simulink model "Demo_PreScanCarSim3D_FMU_cs"  (Simulink 8.6)
settings: Solver=ode5  SolverMode=SingleTasking  StartTime=0.0  StopTime=68  FixedStep=1/1000  RelTol=1e-3
PreLoadFcn:
  | mbxruntime.callbacks.PreLoadFcn(bdroot);
  | check_NUTS_defined;
  | 
  | assignin('base',['model_closed_' bdroot],false);
PostLoadFcn:
  | mbxruntime.callbacks.PostLoadFcn(bdroot);
InitFcn:
  | mbxruntime.callbacks.InitFcn(bdroot);
StartFcn:
  | mbxruntime.callbacks.StartFcn(bdroot);
StopFcn:
  | mbxruntime.callbacks.StopFcn(bdroot);
undefined symbols (not defined in the file or in its folder): DiscIntNeverNeededParam, mbxruntime, tabledata, warningInitialVelocity, x0, x_ini_VRML, y_ini_VRML, z_ini_VRML
libraries: PreScanSimulinkLibrary x15, simulink_extras x8, simulink x5, PreScanCarSimLibrary x1, fmu_cs_lib x1
(part 5 of 11)

== system Demo_PreScanCarSim3D_FMU_cs/VISUCasingLights_TrafficLightRoadSideNL_1/ENABLED/Actuator ==
  VISUCasingLights_TrafficLightRoadSideNL_1 : Inport  Tag=inport/VisuCasingLights  SampleTime=50/1000  BusOutputAsStruct=on
  DemuxVisuLights : Demux  Outputs=3
  LimiterVisuLights : Saturate  UpperLimit=1  LowerLimit=0
  visu_Green [-] : S-Function  FunctionName=sfun_MaterialColorSelector  Parameters=mbxruntime.parameters.convert(UniqueID), mbxruntime.parameters.convert(ColorsObjectQuery), mbxruntime.parameters.convert(Colors),tabledata, TimeStep  SFunctionDeploymentMode=off  EnableBusSupport=off  mask(PreScan Sink Block: VisuTrafficLight){UniqueID=2553, ColorsObjectQuery=child:name=TrafficLightRoadSideNL_1.Casing.LightGreen, Colors=[5   32   25  255    0   64   50  255    0   64   50  255    0    0    0  255; 0   45   34  255    0   45   34  255    0   45   34  255   30  306  240  255], TimeStep=50/1000}
      mask prompts: UniqueID "Parent Unique Identifier"; ColorsObjectQuery "Query for Color Object"; Colors "Matrix of colors"; TimeStep "Simulink time step"
      mask help:
      | The VisuTrafficLight block provides a way to animate traffic lights: switch on and off individual lights.
      |
      | For more information, please click Help.
      mask init:
      | [tabledata] = mbxruntime.parameters.table(UniqueID,ColorsObjectQuery,Colors);
      mask Help: eval('openHelp(731)')
      mask Display: image(imread('TrafficLightCasing.png'))
  visu_Orange [-] : S-Function  FunctionName=sfun_MaterialColorSelector  Parameters=mbxruntime.parameters.convert(UniqueID), mbxruntime.parameters.convert(ColorsObjectQuery), mbxruntime.parameters.convert(Colors),tabledata, TimeStep  SFunctionDeploymentMode=off  EnableBusSupport=off  mask(PreScan Sink Block: VisuTrafficLight){UniqueID=2553, ColorsObjectQuery=child:name=TrafficLightRoadSideNL_1.Casing.LightOrange, Colors=[32   25    5  255   64   48    5  255   64   54    5  255    0    0    0  255; 45   34    0  255   45   34    0  255   45   34    0  255  306  229    5  255], TimeStep=50/1000}
      mask prompts: UniqueID "Parent Unique Identifier"; ColorsObjectQuery "Query for Color Object"; Colors "Matrix of colors"; TimeStep "Simulink time step"
      mask help:
      | The VisuTrafficLight block provides a way to animate traffic lights: switch on and off individual lights.
      |
      | For more information, please click Help.
      mask init:
      | [tabledata] = mbxruntime.parameters.table(UniqueID,ColorsObjectQuery,Colors);
      mask Help: eval('openHelp(731)')
      mask Display: image(imread('TrafficLightCasing.png'))
  visu_Red [-] : S-Function  FunctionName=sfun_MaterialColorSelector  Parameters=mbxruntime.parameters.convert(UniqueID), mbxruntime.parameters.convert(ColorsObjectQuery), mbxruntime.parameters.convert(Colors),tabledata, TimeStep  SFunctionDeploymentMode=off  EnableBusSupport=off  mask(PreScan Sink Block: VisuTrafficLight){UniqueID=2553, ColorsObjectQuery=child:name=TrafficLightRoadSideNL_1.Casing.LightRed, Colors=[32    5    5  255   64    5    5  255   64    5    5  255    0    0    0  255; 45    0    0  255   45    0    0  255   45    0    0  255  306   30   30  255], TimeStep=50/1000}
      mask prompts: UniqueID "Parent Unique Identifier"; ColorsObjectQuery "Query for Color Object"; Colors "Matrix of colors"; TimeStep "Simulink time step"
      mask help:
      | The VisuTrafficLight block provides a way to animate traffic lights: switch on and off individual lights.
      |
      | For more information, please click Help.
      mask init:
      | [tabledata] = mbxruntime.parameters.table(UniqueID,ColorsObjectQuery,Colors);
      mask Help: eval('openHelp(731)')
      mask Display: image(imread('TrafficLightCasing.png'))
  wires:
  VISUCasingLights_TrafficLightRoadSideNL_1/1 -> LimiterVisuLights/1
  LimiterVisuLights/1 -> DemuxVisuLights/1
  DemuxVisuLights/1 -> visu_Green [-]/1
  DemuxVisuLights/2 -> visu_Orange [-]/1
  DemuxVisuLights/3 -> visu_Red [-]/1

== system Demo_PreScanCarSim3D_FMU_cs/VISUCasingLights_TrafficLightRoadSideNL_2/ENABLED/Actuator ==
  VISUCasingLights_TrafficLightRoadSideNL_2 : Inport  Tag=inport/VisuCasingLights  SampleTime=50/1000  BusOutputAsStruct=on
  DemuxVisuLights : Demux  Outputs=3
  LimiterVisuLights : Saturate  UpperLimit=1  LowerLimit=0
  visu_Green [-] : S-Function  FunctionName=sfun_MaterialColorSelector  Parameters=mbxruntime.parameters.convert(UniqueID), mbxruntime.parameters.convert(ColorsObjectQuery), mbxruntime.parameters.convert(Colors),tabledata, TimeStep  SFunctionDeploymentMode=off  EnableBusSupport=off  mask(PreScan Sink Block: VisuTrafficLight){UniqueID=2554, ColorsObjectQuery=child:name=TrafficLightRoadSideNL_2.Casing.LightGreen, Colors=[5   32   25  255    0   64   50  255    0   64   50  255    0    0    0  255; 0   45   34  255    0   45   34  255    0   45   34  255   30  306  240  255], TimeStep=50/1000}
      mask prompts: UniqueID "Parent Unique Identifier"; ColorsObjectQuery "Query for Color Object"; Colors "Matrix of colors"; TimeStep "Simulink time step"
      mask help:
      | The VisuTrafficLight block provides a way to animate traffic lights: switch on and off individual lights.
      |
      | For more information, please click Help.
      mask init:
      | [tabledata] = mbxruntime.parameters.table(UniqueID,ColorsObjectQuery,Colors);
      mask Help: eval('openHelp(731)')
      mask Display: image(imread('TrafficLightCasing.png'))
  visu_Orange [-] : S-Function  FunctionName=sfun_MaterialColorSelector  Parameters=mbxruntime.parameters.convert(UniqueID), mbxruntime.parameters.convert(ColorsObjectQuery), mbxruntime.parameters.convert(Colors),tabledata, TimeStep  SFunctionDeploymentMode=off  EnableBusSupport=off  mask(PreScan Sink Block: VisuTrafficLight){UniqueID=2554, ColorsObjectQuery=child:name=TrafficLightRoadSideNL_2.Casing.LightOrange, Colors=[32   25    5  255   64   48    5  255   64   54    5  255    0    0    0  255; 45   34    0  255   45   34    0  255   45   34    0  255  306  229    5  255], TimeStep=50/1000}
      mask prompts: UniqueID "Parent Unique Identifier"; ColorsObjectQuery "Query for Color Object"; Colors "Matrix of colors"; TimeStep "Simulink time step"
      mask help:
      | The VisuTrafficLight block provides a way to animate traffic lights: switch on and off individual lights.
      |
      | For more information, please click Help.
      mask init:
      | [tabledata] = mbxruntime.parameters.table(UniqueID,ColorsObjectQuery,Colors);
      mask Help: eval('openHelp(731)')
      mask Display: image(imread('TrafficLightCasing.png'))
  visu_Red [-] : S-Function  FunctionName=sfun_MaterialColorSelector  Parameters=mbxruntime.parameters.convert(UniqueID), mbxruntime.parameters.convert(ColorsObjectQuery), mbxruntime.parameters.convert(Colors),tabledata, TimeStep  SFunctionDeploymentMode=off  EnableBusSupport=off  mask(PreScan Sink Block: VisuTrafficLight){UniqueID=2554, ColorsObjectQuery=child:name=TrafficLightRoadSideNL_2.Casing.LightRed, Colors=[32    5    5  255   64    5    5  255   64    5    5  255    0    0    0  255; 45    0    0  255   45    0    0  255   45    0    0  255  306   30   30  255], TimeStep=50/1000}
      mask prompts: UniqueID "Parent Unique Identifier"; ColorsObjectQuery "Query for Color Object"; Colors "Matrix of colors"; TimeStep "Simulink time step"
      mask help:
      | The VisuTrafficLight block provides a way to animate traffic lights: switch on and off individual lights.
      |
      | For more information, please click Help.
      mask init:
      | [tabledata] = mbxruntime.parameters.table(UniqueID,ColorsObjectQuery,Colors);
      mask Help: eval('openHelp(731)')
      mask Display: image(imread('TrafficLightCasing.png'))
  wires:
  VISUCasingLights_TrafficLightRoadSideNL_2/1 -> LimiterVisuLights/1
  LimiterVisuLights/1 -> DemuxVisuLights/1
  DemuxVisuLights/1 -> visu_Green [-]/1
  DemuxVisuLights/2 -> visu_Orange [-]/1
  DemuxVisuLights/3 -> visu_Red [-]/1

== system Demo_PreScanCarSim3D_FMU_cs/VISUCasingLights_TrafficLightRoadSideNL_3/ENABLED/Actuator ==
  VISUCasingLights_TrafficLightRoadSideNL_3 : Inport  Tag=inport/VisuCasingLights  SampleTime=50/1000  BusOutputAsStruct=on
  DemuxVisuLights : Demux  Outputs=3
  LimiterVisuLights : Saturate  UpperLimit=1  LowerLimit=0
  visu_Green [-] : S-Function  FunctionName=sfun_MaterialColorSelector  Parameters=mbxruntime.parameters.convert(UniqueID), mbxruntime.parameters.convert(ColorsObjectQuery), mbxruntime.parameters.convert(Colors),tabledata, TimeStep  SFunctionDeploymentMode=off  EnableBusSupport=off  mask(PreScan Sink Block: VisuTrafficLight){UniqueID=2555, ColorsObjectQuery=child:name=TrafficLightRoadSideNL_3.Casing.LightGreen, Colors=[5   32   25  255    0   64   50  255    0   64   50  255    0    0    0  255; 0   45   34  255    0   45   34  255    0   45   34  255   30  306  240  255], TimeStep=50/1000}
      mask prompts: UniqueID "Parent Unique Identifier"; ColorsObjectQuery "Query for Color Object"; Colors "Matrix of colors"; TimeStep "Simulink time step"
      mask help:
      | The VisuTrafficLight block provides a way to animate traffic lights: switch on and off individual lights.
      |
      | For more information, please click Help.
      mask init:
      | [tabledata] = mbxruntime.parameters.table(UniqueID,ColorsObjectQuery,Colors);
      mask Help: eval('openHelp(731)')
      mask Display: image(imread('TrafficLightCasing.png'))
  visu_Orange [-] : S-Function  FunctionName=sfun_MaterialColorSelector  Parameters=mbxruntime.parameters.convert(UniqueID), mbxruntime.parameters.convert(ColorsObjectQuery), mbxruntime.parameters.convert(Colors),tabledata, TimeStep  SFunctionDeploymentMode=off  EnableBusSupport=off  mask(PreScan Sink Block: VisuTrafficLight){UniqueID=2555, ColorsObjectQuery=child:name=TrafficLightRoadSideNL_3.Casing.LightOrange, Colors=[32   25    5  255   64   48    5  255   64   54    5  255    0    0    0  255; 45   34    0  255   45   34    0  255   45   34    0  255  306  229    5  255], TimeStep=50/1000}
      mask prompts: UniqueID "Parent Unique Identifier"; ColorsObjectQuery "Query for Color Object"; Colors "Matrix of colors"; TimeStep "Simulink time step"
      mask help:
      | The VisuTrafficLight block provides a way to animate traffic lights: switch on and off individual lights.
      |
      | For more information, please click Help.
      mask init:
      | [tabledata] = mbxruntime.parameters.table(UniqueID,ColorsObjectQuery,Colors);
      mask Help: eval('openHelp(731)')
      mask Display: image(imread('TrafficLightCasing.png'))
  visu_Red [-] : S-Function  FunctionName=sfun_MaterialColorSelector  Parameters=mbxruntime.parameters.convert(UniqueID), mbxruntime.parameters.convert(ColorsObjectQuery), mbxruntime.parameters.convert(Colors),tabledata, TimeStep  SFunctionDeploymentMode=off  EnableBusSupport=off  mask(PreScan Sink Block: VisuTrafficLight){UniqueID=2555, ColorsObjectQuery=child:name=TrafficLightRoadSideNL_3.Casing.LightRed, Colors=[32    5    5  255   64    5    5  255   64    5    5  255    0    0    0  255; 45    0    0  255   45    0    0  255   45    0    0  255  306   30   30  255], TimeStep=50/1000}
      mask prompts: UniqueID "Parent Unique Identifier"; ColorsObjectQuery "Query for Color Object"; Colors "Matrix of colors"; TimeStep "Simulink time step"
      mask help:
      | The VisuTrafficLight block provides a way to animate traffic lights: switch on and off individual lights.
      |
      | For more information, please click Help.
      mask init:
      | [tabledata] = mbxruntime.parameters.table(UniqueID,ColorsObjectQuery,Colors);
      mask Help: eval('openHelp(731)')
      mask Display: image(imread('TrafficLightCasing.png'))
  wires:
  VISUCasingLights_TrafficLightRoadSideNL_3/1 -> LimiterVisuLights/1
  LimiterVisuLights/1 -> DemuxVisuLights/1
  DemuxVisuLights/1 -> visu_Green [-]/1
  DemuxVisuLights/2 -> visu_Orange [-]/1
  DemuxVisuLights/3 -> visu_Red [-]/1

== system Demo_PreScanCarSim3D_FMU_cs/VISUCasingLights_TrafficLightRoadSideNL_5/ENABLED/Actuator ==
  VISUCasingLights_TrafficLightRoadSideNL_5 : Inport  Tag=inport/VisuCasingLights  SampleTime=50/1000  BusOutputAsStruct=on
  DemuxVisuLights : Demux  Outputs=3
  LimiterVisuLights : Saturate  UpperLimit=1  LowerLimit=0
  visu_Green [-] : S-Function  FunctionName=sfun_MaterialColorSelector  Parameters=mbxruntime.parameters.convert(UniqueID), mbxruntime.parameters.convert(ColorsObjectQuery), mbxruntime.parameters.convert(Colors),tabledata, TimeStep  SFunctionDeploymentMode=off  EnableBusSupport=off  mask(PreScan Sink Block: VisuTrafficLight){UniqueID=2557, ColorsObjectQuery=child:name=TrafficLightRoadSideNL_5.Casing.LightGreen, Colors=[5   32   25  255    0   64   50  255    0   64   50  255    0    0    0  255; 0   45   34  255    0   45   34  255    0   45   34  255   30  306  240  255], TimeStep=50/1000}
      mask prompts: UniqueID "Parent Unique Identifier"; ColorsObjectQuery "Query for Color Object"; Colors "Matrix of colors"; TimeStep "Simulink time step"
      mask help:
      | The VisuTrafficLight block provides a way to animate traffic lights: switch on and off individual lights.
      |
      | For more information, please click Help.
      mask init:
      | [tabledata] = mbxruntime.parameters.table(UniqueID,ColorsObjectQuery,Colors);
      mask Help: eval('openHelp(731)')
      mask Display: image(imread('TrafficLightCasing.png'))
  visu_Orange [-] : S-Function  FunctionName=sfun_MaterialColorSelector  Parameters=mbxruntime.parameters.convert(UniqueID), mbxruntime.parameters.convert(ColorsObjectQuery), mbxruntime.parameters.convert(Colors),tabledata, TimeStep  SFunctionDeploymentMode=off  EnableBusSupport=off  mask(PreScan Sink Block: VisuTrafficLight){UniqueID=2557, ColorsObjectQuery=child:name=TrafficLightRoadSideNL_5.Casing.LightOrange, Colors=[32   25    5  255   64   48    5  255   64   54    5  255    0    0    0  255; 45   34    0  255   45   34    0  255   45   34    0  255  306  229    5  255], TimeStep=50/1000}
      mask prompts: UniqueID "Parent Unique Identifier"; ColorsObjectQuery "Query for Color Object"; Colors "Matrix of colors"; TimeStep "Simulink time step"
      mask help:
      | The VisuTrafficLight block provides a way to animate traffic lights: switch on and off individual lights.
      |
      | For more information, please click Help.
      mask init:
      | [tabledata] = mbxruntime.parameters.table(UniqueID,ColorsObjectQuery,Colors);
      mask Help: eval('openHelp(731)')
      mask Display: image(imread('TrafficLightCasing.png'))
  visu_Red [-] : S-Function  FunctionName=sfun_MaterialColorSelector  Parameters=mbxruntime.parameters.convert(UniqueID), mbxruntime.parameters.convert(ColorsObjectQuery), mbxruntime.parameters.convert(Colors),tabledata, TimeStep  SFunctionDeploymentMode=off  EnableBusSupport=off  mask(PreScan Sink Block: VisuTrafficLight){UniqueID=2557, ColorsObjectQuery=child:name=TrafficLightRoadSideNL_5.Casing.LightRed, Colors=[32    5    5  255   64    5    5  255   64    5    5  255    0    0    0  255; 45    0    0  255   45    0    0  255   45    0    0  255  306   30   30  255], TimeStep=50/1000}
      mask prompts: UniqueID "Parent Unique Identifier"; ColorsObjectQuery "Query for Color Object"; Colors "Matrix of colors"; TimeStep "Simulink time step"
      mask help:
      | The VisuTrafficLight block provides a way to animate traffic lights: switch on and off individual lights.
      |
      | For more information, please click Help.
      mask init:
      | [tabledata] = mbxruntime.parameters.table(UniqueID,ColorsObjectQuery,Colors);
      mask Help: eval('openHelp(731)')
      mask Display: image(imread('TrafficLightCasing.png'))
  wires:
  VISUCasingLights_TrafficLightRoadSideNL_5/1 -> LimiterVisuLights/1
  LimiterVisuLights/1 -> DemuxVisuLights/1
  DemuxVisuLights/1 -> visu_Green [-]/1
  DemuxVisuLights/2 -> visu_Orange [-]/1
  DemuxVisuLights/3 -> visu_Red [-]/1

== system Demo_PreScanCarSim3D_FMU_cs/VISUCasingLights_TrafficLightRoadSideNL_6/ENABLED/Actuator ==
  VISUCasingLights_TrafficLightRoadSideNL_6 : Inport  Tag=inport/VisuCasingLights  SampleTime=50/1000  BusOutputAsStruct=on
  DemuxVisuLights : Demux  Outputs=3
  LimiterVisuLights : Saturate  UpperLimit=1  LowerLimit=0
  visu_Green [-] : S-Function  FunctionName=sfun_MaterialColorSelector  Parameters=mbxruntime.parameters.convert(UniqueID), mbxruntime.parameters.convert(ColorsObjectQuery), mbxruntime.parameters.convert(Colors),tabledata, TimeStep  SFunctionDeploymentMode=off  EnableBusSupport=off  mask(PreScan Sink Block: VisuTrafficLight){UniqueID=2558, ColorsObjectQuery=child:name=TrafficLightRoadSideNL_6.Casing.LightGreen, Colors=[5   32   25  255    0   64   50  255    0   64   50  255    0    0    0  255; 0   45   34  255    0   45   34  255    0   45   34  255   30  306  240  255], TimeStep=50/1000}
      mask prompts: UniqueID "Parent Unique Identifier"; ColorsObjectQuery "Query for Color Object"; Colors "Matrix of colors"; TimeStep "Simulink time step"
      mask help:
      | The VisuTrafficLight block provides a way to animate traffic lights: switch on and off individual lights.
      |
      | For more information, please click Help.
      mask init:
      | [tabledata] = mbxruntime.parameters.table(UniqueID,ColorsObjectQuery,Colors);
      mask Help: eval('openHelp(731)')
      mask Display: image(imread('TrafficLightCasing.png'))
  visu_Orange [-] : S-Function  FunctionName=sfun_MaterialColorSelector  Parameters=mbxruntime.parameters.convert(UniqueID), mbxruntime.parameters.convert(ColorsObjectQuery), mbxruntime.parameters.convert(Colors),tabledata, TimeStep  SFunctionDeploymentMode=off  EnableBusSupport=off  mask(PreScan Sink Block: VisuTrafficLight){UniqueID=2558, ColorsObjectQuery=child:name=TrafficLightRoadSideNL_6.Casing.LightOrange, Colors=[32   25    5  255   64   48    5  255   64   54    5  255    0    0    0  255; 45   34    0  255   45   34    0  255   45   34    0  255  306  229    5  255], TimeStep=50/1000}
      mask prompts: UniqueID "Parent Unique Identifier"; ColorsObjectQuery "Query for Color Object"; Colors "Matrix of colors"; TimeStep "Simulink time step"
      mask help:
      | The VisuTrafficLight block provides a way to animate traffic lights: switch on and off individual lights.
      |
      | For more information, please click Help.
      mask init:
      | [tabledata] = mbxruntime.parameters.table(UniqueID,ColorsObjectQuery,Colors);
      mask Help: eval('openHelp(731)')
      mask Display: image(imread('TrafficLightCasing.png'))
  visu_Red [-] : S-Function  FunctionName=sfun_MaterialColorSelector  Parameters=mbxruntime.parameters.convert(UniqueID), mbxruntime.parameters.convert(ColorsObjectQuery), mbxruntime.parameters.convert(Colors),tabledata, TimeStep  SFunctionDeploymentMode=off  EnableBusSupport=off  mask(PreScan Sink Block: VisuTrafficLight){UniqueID=2558, ColorsObjectQuery=child:name=TrafficLightRoadSideNL_6.Casing.LightRed, Colors=[32    5    5  255   64    5    5  255   64    5    5  255    0    0    0  255; 45    0    0  255   45    0    0  255   45    0    0  255  306   30   30  255], TimeStep=50/1000}
      mask prompts: UniqueID "Parent Unique Identifier"; ColorsObjectQuery "Query for Color Object"; Colors "Matrix of colors"; TimeStep "Simulink time step"
      mask help:
      | The VisuTrafficLight block provides a way to animate traffic lights: switch on and off individual lights.
      |
      | For more information, please click Help.
      mask init:
      | [tabledata] = mbxruntime.parameters.table(UniqueID,ColorsObjectQuery,Colors);
      mask Help: eval('openHelp(731)')
      mask Display: image(imread('TrafficLightCasing.png'))
  wires:
  VISUCasingLights_TrafficLightRoadSideNL_6/1 -> LimiterVisuLights/1
  LimiterVisuLights/1 -> DemuxVisuLights/1
  DemuxVisuLights/1 -> visu_Green [-]/1
  DemuxVisuLights/2 -> visu_Orange [-]/1
  DemuxVisuLights/3 -> visu_Red [-]/1

== system Demo_PreScanCarSim3D_FMU_cs/VISUCasingLights_TrafficLightRoadSideNL_7/ENABLED/Actuator ==
  VISUCasingLights_TrafficLightRoadSideNL_7 : Inport  Tag=inport/VisuCasingLights  SampleTime=50/1000  BusOutputAsStruct=on
  DemuxVisuLights : Demux  Outputs=3
  LimiterVisuLights : Saturate  UpperLimit=1  LowerLimit=0
  visu_Green [-] : S-Function  FunctionName=sfun_MaterialColorSelector  Parameters=mbxruntime.parameters.convert(UniqueID), mbxruntime.parameters.convert(ColorsObjectQuery), mbxruntime.parameters.convert(Colors),tabledata, TimeStep  SFunctionDeploymentMode=off  EnableBusSupport=off  mask(PreScan Sink Block: VisuTrafficLight){UniqueID=2559, ColorsObjectQuery=child:name=TrafficLightRoadSideNL_7.Casing.LightGreen, Colors=[5   32   25  255    0   64   50  255    0   64   50  255    0    0    0  255; 0   45   34  255    0   45   34  255    0   45   34  255   30  306  240  255], TimeStep=50/1000}
      mask prompts: UniqueID "Parent Unique Identifier"; ColorsObjectQuery "Query for Color Object"; Colors "Matrix of colors"; TimeStep "Simulink time step"
      mask help:
      | The VisuTrafficLight block provides a way to animate traffic lights: switch on and off individual lights.
      |
      | For more information, please click Help.
      mask init:
      | [tabledata] = mbxruntime.parameters.table(UniqueID,ColorsObjectQuery,Colors);
      mask Help: eval('openHelp(731)')
      mask Display: image(imread('TrafficLightCasing.png'))
  visu_Orange [-] : S-Function  FunctionName=sfun_MaterialColorSelector  Parameters=mbxruntime.parameters.convert(UniqueID), mbxruntime.parameters.convert(ColorsObjectQuery), mbxruntime.parameters.convert(Colors),tabledata, TimeStep  SFunctionDeploymentMode=off  EnableBusSupport=off  mask(PreScan Sink Block: VisuTrafficLight){UniqueID=2559, ColorsObjectQuery=child:name=TrafficLightRoadSideNL_7.Casing.LightOrange, Colors=[32   25    5  255   64   48    5  255   64   54    5  255    0    0    0  255; 45   34    0  255   45   34    0  255   45   34    0  255  306  229    5  255], TimeStep=50/1000}
      mask prompts: UniqueID "Parent Unique Identifier"; ColorsObjectQuery "Query for Color Object"; Colors "Matrix of colors"; TimeStep "Simulink time step"
      mask help:
      | The VisuTrafficLight block provides a way to animate traffic lights: switch on and off individual lights.
      |
      | For more information, please click Help.
      mask init:
      | [tabledata] = mbxruntime.parameters.table(UniqueID,ColorsObjectQuery,Colors);
      mask Help: eval('openHelp(731)')
      mask Display: image(imread('TrafficLightCasing.png'))
  visu_Red [-] : S-Function  FunctionName=sfun_MaterialColorSelector  Parameters=mbxruntime.parameters.convert(UniqueID), mbxruntime.parameters.convert(ColorsObjectQuery), mbxruntime.parameters.convert(Colors),tabledata, TimeStep  SFunctionDeploymentMode=off  EnableBusSupport=off  mask(PreScan Sink Block: VisuTrafficLight){UniqueID=2559, ColorsObjectQuery=child:name=TrafficLightRoadSideNL_7.Casing.LightRed, Colors=[32    5    5  255   64    5    5  255   64    5    5  255    0    0    0  255; 45    0    0  255   45    0    0  255   45    0    0  255  306   30   30  255], TimeStep=50/1000}
      mask prompts: UniqueID "Parent Unique Identifier"; ColorsObjectQuery "Query for Color Object"; Colors "Matrix of colors"; TimeStep "Simulink time step"
      mask help:
      | The VisuTrafficLight block provides a way to animate traffic lights: switch on and off individual lights.
      |
      | For more information, please click Help.
      mask init:
      | [tabledata] = mbxruntime.parameters.table(UniqueID,ColorsObjectQuery,Colors);
      mask Help: eval('openHelp(731)')
      mask Display: image(imread('TrafficLightCasing.png'))
  wires:
  VISUCasingLights_TrafficLightRoadSideNL_7/1 -> LimiterVisuLights/1
  LimiterVisuLights/1 -> DemuxVisuLights/1
  DemuxVisuLights/1 -> visu_Green [-]/1
  DemuxVisuLights/2 -> visu_Orange [-]/1
  DemuxVisuLights/3 -> visu_Red [-]/1

== system Demo_PreScanCarSim3D_FMU_cs/VISUMatrixSignLights_HighwayOverhang_1/ENABLED/Actuator ==
  VISUMatrixSignLights_HighwayOverhang_1 : Inport  Tag=inport/VisuMatrixSignLights  SampleTime=50/1000  BusOutputAsStruct=on
  DemuxVisuLights : Demux  Outputs=16
  LimiterVisuLights : Saturate  UpperLimit=1  LowerLimit=0
  visu_MatrixSign_1_Light_1 : S-Function  FunctionName=sfun_MaterialColorSelector  Parameters=mbxruntime.parameters.convert(UniqueID), mbxruntime.parameters.convert(ColorsObjectQuery), mbxruntime.parameters.convert(Colors),tabledata, TimeStep  SFunctionDeploymentMode=off  EnableBusSupport=off  mask(PreScan Sink Block: VisuMatrixSignLights){UniqueID=1876, ColorsObjectQuery=child:name=hcn/child:name=MatrixSign_1/child:name=HighwayOverhang_1.MatrixSign_1.OrangeLightUpperLeft, Colors=[32   25    5  255   64   48    5  255   64   54    5  255    0    0    0  255; 45   34    0  255   45   34    0  255   45   34    0  255  306  229    5  255], TimeStep=50/1000}
      mask prompts: UniqueID "Parent Unique Identifier"; ColorsObjectQuery "Query for Color Object"; Colors "Matrix of colors"; TimeStep "Simulink time step"
      mask help:
      | The VisuMatrixSignLights block provides a way to switch the lights on the matrix sign board on or off
      |
      | For more information, please click Help.
      mask init:
      | [tabledata] = mbxruntime.parameters.table(UniqueID,ColorsObjectQuery,Colors);
      mask Help: eval('openHelp(732)')
      mask Display: image(imread('RearLight.png'))
  visu_MatrixSign_1_Light_2 : S-Function  FunctionName=sfun_MaterialColorSelector  Parameters=mbxruntime.parameters.convert(UniqueID), mbxruntime.parameters.convert(ColorsObjectQuery), mbxruntime.parameters.convert(Colors),tabledata, TimeStep  SFunctionDeploymentMode=off  EnableBusSupport=off  mask(PreScan Sink Block: VisuMatrixSignLights){UniqueID=1876, ColorsObjectQuery=child:name=hcn/child:name=MatrixSign_1/child:name=HighwayOverhang_1.MatrixSign_1.OrangeLightUpperRight, Colors=[32   25    5  255   64   48    5  255   64   54    5  255    0    0    0  255; 45   34    0  255   45   34    0  255   45   34    0  255  306  229    5  255], TimeStep=50/1000}
      mask prompts: UniqueID "Parent Unique Identifier"; ColorsObjectQuery "Query for Color Object"; Colors "Matrix of colors"; TimeStep "Simulink time step"
      mask help:
      | The VisuMatrixSignLights block provides a way to switch the lights on the matrix sign board on or off
      |
      | For more information, please click Help.
      mask init:
      | [tabledata] = mbxruntime.parameters.table(UniqueID,ColorsObjectQuery,Colors);
      mask Help: eval('openHelp(732)')
      mask Display: image(imread('RearLight.png'))
  visu_MatrixSign_1_Light_3 : S-Function  FunctionName=sfun_MaterialColorSelector  Parameters=mbxruntime.parameters.convert(UniqueID), mbxruntime.parameters.convert(ColorsObjectQuery), mbxruntime.parameters.convert(Colors),tabledata, TimeStep  SFunctionDeploymentMode=off  EnableBusSupport=off  mask(PreScan Sink Block: VisuMatrixSignLights){UniqueID=1876, ColorsObjectQuery=child:name=hcn/child:name=MatrixSign_1/child:name=HighwayOverhang_1.MatrixSign_1.OrangeLightLowerLeft, Colors=[32   25    5  255   64   48    5  255   64   54    5  255    0    0    0  255; 45   34    0  255   45   34    0  255   45   34    0  255  306  229    5  255], TimeStep=50/1000}
      mask prompts: UniqueID "Parent Unique Identifier"; ColorsObjectQuery "Query for Color Object"; Colors "Matrix of colors"; TimeStep "Simulink time step"
      mask help:
      | The VisuMatrixSignLights block provides a way to switch the lights on the matrix sign board on or off
      |
      | For more information, please click Help.
      mask init:
      | [tabledata] = mbxruntime.parameters.table(UniqueID,ColorsObjectQuery,Colors);
      mask Help: eval('openHelp(732)')
      mask Display: image(imread('RearLight.png'))
  visu_MatrixSign_1_Light_4 : S-Function  FunctionName=sfun_MaterialColorSelector  Parameters=mbxruntime.parameters.convert(UniqueID), mbxruntime.parameters.convert(ColorsObjectQuery), mbxruntime.parameters.convert(Colors),tabledata, TimeStep  SFunctionDeploymentMode=off  EnableBusSupport=off  mask(PreScan Sink Block: VisuMatrixSignLights){UniqueID=1876, ColorsObjectQuery=child:name=hcn/child:name=MatrixSign_1/child:name=HighwayOverhang_1.MatrixSign_1.OrangeLightLowerRight, Colors=[32   25    5  255   64   48    5  255   64   54    5  255    0    0    0  255; 45   34    0  255   45   34    0  255   45   34    0  255  306  229    5  255], TimeStep=50/1000}
      mask prompts: UniqueID "Parent Unique Identifier"; ColorsObjectQuery "Query for Color Object"; Colors "Matrix of colors"; TimeStep "Simulink time step"
      mask help:
      | The VisuMatrixSignLights block provides a way to switch the lights on the matrix sign board on or off
      |
      | For more information, please click Help.
      mask init:
      | [tabledata] = mbxruntime.parameters.table(UniqueID,ColorsObjectQuery,Colors);
      mask Help: eval('openHelp(732)')
      mask Display: image(imread('RearLight.png'))
  visu_MatrixSign_2_Light_1 : S-Function  FunctionName=sfun_MaterialColorSelector  Parameters=mbxruntime.parameters.convert(UniqueID), mbxruntime.parameters.convert(ColorsObjectQuery), mbxruntime.parameters.convert(Colors),tabledata, TimeStep  SFunctionDeploymentMode=off  EnableBusSupport=off  mask(PreScan Sink Block: VisuMatrixSignLights){UniqueID=1876, ColorsObjectQuery=child:name=hcn/child:name=MatrixSign_2/child:name=HighwayOverhang_1.MatrixSign_2.OrangeLightUpperLeft, Colors=[32   25    5  255   64   48    5  255   64   54    5  255    0    0    0  255; 45   34    0  255   45   34    0  255   45   34    0  255  306  229    5  255], TimeStep=50/1000}
      mask prompts: UniqueID "Parent Unique Identifier"; ColorsObjectQuery "Query for Color Object"; Colors "Matrix of colors"; TimeStep "Simulink time step"
      mask help:
      | The VisuMatrixSignLights block provides a way to switch the lights on the matrix sign board on or off
      |
      | For more information, please click Help.
      mask init:
      | [tabledata] = mbxruntime.parameters.table(UniqueID,ColorsObjectQuery,Colors);
      mask Help: eval('openHelp(732)')
      mask Display: image(imread('RearLight.png'))
  visu_MatrixSign_2_Light_2 : S-Function  FunctionName=sfun_MaterialColorSelector  Parameters=mbxruntime.parameters.convert(UniqueID), mbxruntime.parameters.convert(ColorsObjectQuery), mbxruntime.parameters.convert(Colors),tabledata, TimeStep  SFunctionDeploymentMode=off  EnableBusSupport=off  mask(PreScan Sink Block: VisuMatrixSignLights){UniqueID=1876, ColorsObjectQuery=child:name=hcn/child:name=MatrixSign_2/child:name=HighwayOverhang_1.MatrixSign_2.OrangeLightUpperRight, Colors=[32   25    5  255   64   48    5  255   64   54    5  255    0    0    0  255; 45   34    0  255   45   34    0  255   45   34    0  255  306  229    5  255], TimeStep=50/1000}
      mask prompts: UniqueID "Parent Unique Identifier"; ColorsObjectQuery "Query for Color Object"; Colors "Matrix of colors"; TimeStep "Simulink time step"
      mask help:
      | The VisuMatrixSignLights block provides a way to switch the lights on the matrix sign board on or off
      |
      | For more information, please click Help.
      mask init:
      | [tabledata] = mbxruntime.parameters.table(UniqueID,ColorsObjectQuery,Colors);
      mask Help: eval('openHelp(732)')
      mask Display: image(imread('RearLight.png'))
  visu_MatrixSign_2_Light_3 : S-Function  FunctionName=sfun_MaterialColorSelector  Parameters=mbxruntime.parameters.convert(UniqueID), mbxruntime.parameters.convert(ColorsObjectQuery), mbxruntime.parameters.convert(Colors),tabledata, TimeStep  SFunctionDeploymentMode=off  EnableBusSupport=off  mask(PreScan Sink Block: VisuMatrixSignLights){UniqueID=1876, ColorsObjectQuery=child:name=hcn/child:name=MatrixSign_2/child:name=HighwayOverhang_1.MatrixSign_2.OrangeLightLowerLeft, Colors=[32   25    5  255   64   48    5  255   64   54    5  255    0    0    0  255; 45   34    0  255   45   34    0  255   45   34    0  255  306  229    5  255], TimeStep=50/1000}
      mask prompts: UniqueID "Parent Unique Identifier"; ColorsObjectQuery "Query for Color Object"; Colors "Matrix of colors"; TimeStep "Simulink time step"
      mask help:
      | The VisuMatrixSignLights block provides a way to switch the lights on the matrix sign board on or off
      |
      | For more information, please click Help.
      mask init:
      | [tabledata] = mbxruntime.parameters.table(UniqueID,ColorsObjectQuery,Colors);
      mask Help: eval('openHelp(732)')
      mask Display: image(imread('RearLight.png'))
  visu_MatrixSign_2_Light_4 : S-Function  FunctionName=sfun_MaterialColorSelector  Parameters=mbxruntime.parameters.convert(UniqueID), mbxruntime.parameters.convert(ColorsObjectQuery), mbxruntime.parameters.convert(Colors),tabledata, TimeStep  SFunctionDeploymentMode=off  EnableBusSupport=off  mask(PreScan Sink Block: VisuMatrixSignLights){UniqueID=1876, ColorsObjectQuery=child:name=hcn/child:name=MatrixSign_2/child:name=HighwayOverhang_1.MatrixSign_2.OrangeLightLowerRight, Colors=[32   25    5  255   64   48    5  255   64   54    5  255    0    0    0  255; 45   34    0  255   45   34    0  255   45   34    0  255  306  229    5  255], TimeStep=50/1000}
      mask prompts: UniqueID "Parent Unique Identifier"; ColorsObjectQuery "Query for Color Object"; Colors "Matrix of colors"; TimeStep "Simulink time step"
      mask help:
      | The VisuMatrixSignLights block provides a way to switch the lights on the matrix sign board on or off
      |
      | For more information, please click Help.
      mask init:
      | [tabledata] = mbxruntime.parameters.table(UniqueID,ColorsObjectQuery,Colors);
      mask Help: eval('openHelp(732)')
      mask Display: image(imread('RearLight.png'))
  visu_MatrixSign_3_Light_1 : S-Function  FunctionName=sfun_MaterialColorSelector  Parameters=mbxruntime.parameters.convert(UniqueID), mbxruntime.parameters.convert(ColorsObjectQuery), mbxruntime.parameters.convert(Colors),tabledata, TimeStep  SFunctionDeploymentMode=off  EnableBusSupport=off  mask(PreScan Sink Block: VisuMatrixSignLights){UniqueID=1876, ColorsObjectQuery=child:name=hcn/child:name=MatrixSign_3/child:name=HighwayOverhang_1.MatrixSign_3.OrangeLightUpperLeft, Colors=[32   25    5  255   64   48    5  255   64   54    5  255    0    0    0  255; 45   34    0  255   45   34    0  255   45   34    0  255  306  229    5  255], TimeStep=50/1000}
      mask prompts: UniqueID "Parent Unique Identifier"; ColorsObjectQuery "Query for Color Object"; Colors "Matrix of colors"; TimeStep "Simulink time step"
      mask help:
      | The VisuMatrixSignLights block provides a way to switch the lights on the matrix sign board on or off
      |
      | For more information, please click Help.
      mask init:
      | [tabledata] = mbxruntime.parameters.table(UniqueID,ColorsObjectQuery,Colors);
      mask Help: eval('openHelp(732)')
      mask Display: image(imread('RearLight.png'))
  visu_MatrixSign_3_Light_2 : S-Function  FunctionName=sfun_MaterialColorSelector  Parameters=mbxruntime.parameters.convert(UniqueID), mbxruntime.parameters.convert(ColorsObjectQuery), mbxruntime.parameters.convert(Colors),tabledata, TimeStep  SFunctionDeploymentMode=off  EnableBusSupport=off  mask(PreScan Sink Block: VisuMatrixSignLights){UniqueID=1876, ColorsObjectQuery=child:name=hcn/child:name=MatrixSign_3/child:name=HighwayOverhang_1.MatrixSign_3.OrangeLightUpperRight, Colors=[32   25    5  255   64   48    5  255   64   54    5  255    0    0    0  255; 45   34    0  255   45   34    0  255   45   34    0  255  306  229    5  255], TimeStep=50/1000}
      mask prompts: UniqueID "Parent Unique Identifier"; ColorsObjectQuery "Query for Color Object"; Colors "Matrix of colors"; TimeStep "Simulink time step"
      mask help:
      | The VisuMatrixSignLights block provides a way to switch the lights on the matrix sign board on or off
      |
      | For more information, please click Help.
      mask init:
      | [tabledata] = mbxruntime.parameters.table(UniqueID,ColorsObjectQuery,Colors);
      mask Help: eval('openHelp(732)')
      mask Display: image(imread('RearLight.png'))
  visu_MatrixSign_3_Light_3 : S-Function  FunctionName=sfun_MaterialColorSelector  Parameters=mbxruntime.parameters.convert(UniqueID), mbxruntime.parameters.convert(ColorsObjectQuery), mbxruntime.parameters.convert(Colors),tabledata, TimeStep  SFunctionDeploymentMode=off  EnableBusSupport=off  mask(PreScan Sink Block: VisuMatrixSignLights){UniqueID=1876, ColorsObjectQuery=child:name=hcn/child:name=MatrixSign_3/child:name=HighwayOverhang_1.MatrixSign_3.OrangeLightLowerLeft, Colors=[32   25    5  255   64   48    5  255   64   54    5  255    0    0    0  255; 45   34    0  255   45   34    0  255   45   34    0  255  306  229    5  255], TimeStep=50/1000}
      mask prompts: UniqueID "Parent Unique Identifier"; ColorsObjectQuery "Query for Color Object"; Colors "Matrix of colors"; TimeStep "Simulink time step"
      mask help:
      | The VisuMatrixSignLights block provides a way to switch the lights on the matrix sign board on or off
      |
      | For more information, please click Help.
      mask init:
      | [tabledata] = mbxruntime.parameters.table(UniqueID,ColorsObjectQuery,Colors);
      mask Help: eval('openHelp(732)')
      mask Display: image(imread('RearLight.png'))
  visu_MatrixSign_3_Light_4 : S-Function  FunctionName=sfun_MaterialColorSelector  Parameters=mbxruntime.parameters.convert(UniqueID), mbxruntime.parameters.convert(ColorsObjectQuery), mbxruntime.parameters.convert(Colors),tabledata, TimeStep  SFunctionDeploymentMode=off  EnableBusSupport=off  mask(PreScan Sink Block: VisuMatrixSignLights){UniqueID=1876, ColorsObjectQuery=child:name=hcn/child:name=MatrixSign_3/child:name=HighwayOverhang_1.MatrixSign_3.OrangeLightLowerRight, Colors=[32   25    5  255   64   48    5  255   64   54    5  255    0    0    0  255; 45   34    0  255   45   34    0  255   45   34    0  255  306  229    5  255], TimeStep=50/1000}
      mask prompts: UniqueID "Parent Unique Identifier"; ColorsObjectQuery "Query for Color Object"; Colors "Matrix of colors"; TimeStep "Simulink time step"
      mask help:
      | The VisuMatrixSignLights block provides a way to switch the lights on the matrix sign board on or off
      |
      | For more information, please click Help.
      mask init:
      | [tabledata] = mbxruntime.parameters.table(UniqueID,ColorsObjectQuery,Colors);
      mask Help: eval('openHelp(732)')
      mask Display: image(imread('RearLight.png'))
  visu_MatrixSign_4_Light_1 : S-Function  FunctionName=sfun_MaterialColorSelector  Parameters=mbxruntime.parameters.convert(UniqueID), mbxruntime.parameters.convert(ColorsObjectQuery), mbxruntime.parameters.convert(Colors),tabledata, TimeStep  SFunctionDeploymentMode=off  EnableBusSupport=off  mask(PreScan Sink Block: VisuMatrixSignLights){UniqueID=1876, ColorsObjectQuery=child:name=hcn/child:name=MatrixSign_4/child:name=HighwayOverhang_1.MatrixSign_4.OrangeLightUpperLeft, Colors=[32   25    5  255   64   48    5  255   64   54    5  255    0    0    0  255; 45   34    0  255   45   34    0  255   45   34    0  255  306  229    5  255], TimeStep=50/1000}
      mask prompts: UniqueID "Parent Unique Identifier"; ColorsObjectQuery "Query for Color Object"; Colors "Matrix of colors"; TimeStep "Simulink time step"
      mask help:
      | The VisuMatrixSignLights block provides a way to switch the lights on the matrix sign board on or off
      |
      | For more information, please click Help.
      mask init:
      | [tabledata] = mbxruntime.parameters.table(UniqueID,ColorsObjectQuery,Colors);
      mask Help: eval('openHelp(732)')
      mask Display: image(imread('RearLight.png'))
  visu_MatrixSign_4_Light_2 : S-Function  FunctionName=sfun_MaterialColorSelector  Parameters=mbxruntime.parameters.convert(UniqueID), mbxruntime.parameters.convert(ColorsObjectQuery), mbxruntime.parameters.convert(Colors),tabledata, TimeStep  SFunctionDeploymentMode=off  EnableBusSupport=off  mask(PreScan Sink Block: VisuMatrixSignLights){UniqueID=1876, ColorsObjectQuery=child:name=hcn/child:name=MatrixSign_4/child:name=HighwayOverhang_1.MatrixSign_4.OrangeLightUpperRight, Colors=[32   25    5  255   64   48    5  255   64   54    5  255    0    0    0  255; 45   34    0  255   45   34    0  255   45   34    0  255  306  229    5  255], TimeStep=50/1000}
      mask prompts: UniqueID "Parent Unique Identifier"; ColorsObjectQuery "Query for Color Object"; Colors "Matrix of colors"; TimeStep "Simulink time step"
      mask help:
      | The VisuMatrixSignLights block provides a way to switch the lights on the matrix sign board on or off
      |
      | For more information, please click Help.
      mask init:
      | [tabledata] = mbxruntime.parameters.table(UniqueID,ColorsObjectQuery,Colors);
      mask Help: eval('openHelp(732)')
      mask Display: image(imread('RearLight.png'))
  visu_MatrixSign_4_Light_3 : S-Function  FunctionName=sfun_MaterialColorSelector  Parameters=mbxruntime.parameters.convert(UniqueID), mbxruntime.parameters.convert(ColorsObjectQuery), mbxruntime.parameters.convert(Colors),tabledata, TimeStep  SFunctionDeploymentMode=off  EnableBusSupport=off  mask(PreScan Sink Block: VisuMatrixSignLights){UniqueID=1876, ColorsObjectQuery=child:name=hcn/child:name=MatrixSign_4/child:name=HighwayOverhang_1.MatrixSign_4.OrangeLightLowerLeft, Colors=[32   25    5  255   64   48    5  255   64   54    5  255    0    0    0  255; 45   34    0  255   45   34    0  255   45   34    0  255  306  229    5  255], TimeStep=50/1000}
      mask prompts: UniqueID "Parent Unique Identifier"; ColorsObjectQuery "Query for Color Object"; Colors "Matrix of colors"; TimeStep "Simulink time step"
      mask help:
      | The VisuMatrixSignLights block provides a way to switch the lights on the matrix sign board on or off
      |
      | For more information, please click Help.
      mask init:
      | [tabledata] = mbxruntime.parameters.table(UniqueID,ColorsObjectQuery,Colors);
      mask Help: eval('openHelp(732)')
      mask Display: image(imread('RearLight.png'))
  visu_MatrixSign_4_Light_4 : S-Function  FunctionName=sfun_MaterialColorSelector  Parameters=mbxruntime.parameters.convert(UniqueID), mbxruntime.parameters.convert(ColorsObjectQuery), mbxruntime.parameters.convert(Colors),tabledata, TimeStep  SFunctionDeploymentMode=off  EnableBusSupport=off  mask(PreScan Sink Block: VisuMatrixSignLights){UniqueID=1876, ColorsObjectQuery=child:name=hcn/child:name=MatrixSign_4/child:name=HighwayOverhang_1.MatrixSign_4.OrangeLightLowerRight, Colors=[32   25    5  255   64   48    5  255   64   54    5  255    0    0    0  255; 45   34    0  255   45   34    0  255   45   34    0  255  306  229    5  255], TimeStep=50/1000}
      mask prompts: UniqueID "Parent Unique Identifier"; ColorsObjectQuery "Query for Color Object"; Colors "Matrix of colors"; TimeStep "Simulink time step"
      mask help:
      | The VisuMatrixSignLights block provides a way to switch the lights on the matrix sign board on or off
      |
      | For more information, please click Help.
      mask init:
      | [tabledata] = mbxruntime.parameters.table(UniqueID,ColorsObjectQuery,Colors);
      mask Help: eval('openHelp(732)')
      mask Display: image(imread('RearLight.png'))
  wires:
  VISUMatrixSignLights_HighwayOverhang_1/1 -> LimiterVisuLights/1
  LimiterVisuLights/1 -> DemuxVisuLights/1
  DemuxVisuLights/1 -> visu_MatrixSign_1_Light_1/1
  DemuxVisuLights/2 -> visu_MatrixSign_1_Light_2/1
  DemuxVisuLights/3 -> visu_MatrixSign_1_Light_3/1
  DemuxVisuLights/4 -> visu_MatrixSign_1_Light_4/1
  DemuxVisuLights/5 -> visu_MatrixSign_2_Light_1/1
  DemuxVisuLights/6 -> visu_MatrixSign_2_Light_2/1
  DemuxVisuLights/7 -> visu_MatrixSign_2_Light_3/1
  DemuxVisuLights/8 -> visu_MatrixSign_2_Light_4/1
  DemuxVisuLights/9 -> visu_MatrixSign_3_Light_1/1
  DemuxVisuLights/10 -> visu_MatrixSign_3_Light_2/1
  DemuxVisuLights/11 -> visu_MatrixSign_3_Light_3/1
  DemuxVisuLights/12 -> visu_MatrixSign_3_Light_4/1
  DemuxVisuLights/13 -> visu_MatrixSign_4_Light_1/1
  DemuxVisuLights/14 -> visu_MatrixSign_4_Light_2/1
  DemuxVisuLights/15 -> visu_MatrixSign_4_Light_3/1
  DemuxVisuLights/16 -> visu_MatrixSign_4_Light_4/1
